simulink model "decoupler_ss"  (R2024a)
settings: Solver=VariableStepAuto  StartTime=0.0  StopTime=30  RelTol=1e-3
values from neighbouring files (symbols this model uses):
  A = [-1.7, -0.25, 0 ... (first row only)    [main.m]
  B = [7, 0 ... (first row only)    [main.m]
  C = [0, 1, 0 ... (first row only)    [main.m]
  F = inv(Bstar)    [decoupling.m]
  K = real(R \ B' * P)    [LQR_own.m]    (also in decoupling.m = Bstar\C_star; main.m = real(inv(R)*B_bar'*P); pole_placement.m = Kbar*T)
  x0 = [1 100 200]'    [main.m]
settings Model: Creator=chint  LastModifiedBy=chint

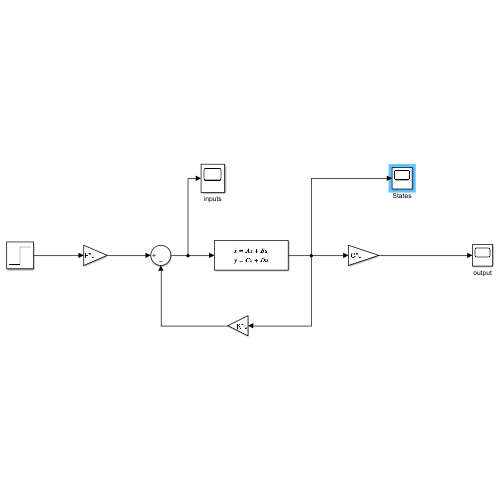
[thumbnail: Simulink's stored preview of the top-level diagram]
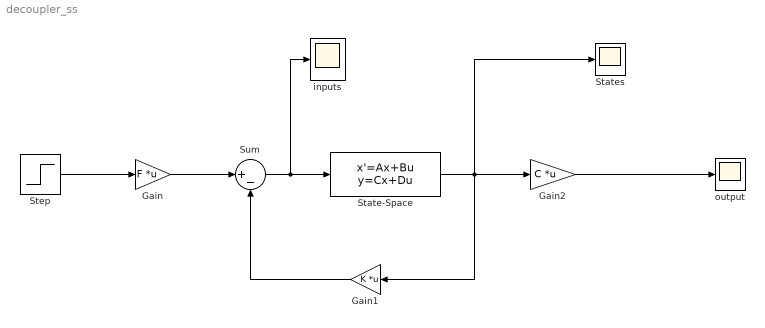
== system decoupler_ss ==
  Gain : Gain  Gain=F  Multiplication=Matrix(K*u)
  Gain1 : Gain  Gain=K  Multiplication=Matrix(K*u)
  Gain2 : Gain  Gain=C  Multiplication=Matrix(K*u)
  State-Space : StateSpace  A=A  B=B  C=eye(3)  D=zeros(3,2)  InitialCondition=x0
  States : Scope
  Step : Step  Before=[0;0]  After=[0;1]  SampleTime=0
  Sum : Sum  Inputs=|+-
  inputs : Scope
  output : Scope
  wires:
  Step/1 -> Gain/1
  Gain/1 -> Sum/1
  Gain1/1 -> Sum/2
  Sum/1 -> inputs/1, State-Space/1
  State-Space/1 -> States/1, Gain2/1, Gain1/1
  Gain2/1 -> output/1
